simulink model "controlP"  (R2021a)
settings: Solver=VariableStepAuto  StartTime=0.0  StopTime=10.0  RelTol=1e-3
libraries: simulink x1
settings Model: Creator=phcs  LastModifiedBy=phcs

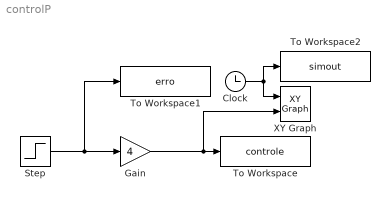
== system controlP ==
  Clock : Clock
  Gain : Gain  Gain=4
  Step : Step  Time=0  SampleTime=0
  To Workspace : ToWorkspace  VariableName=controle  SaveFormat=Timeseries  SampleTime=-1
  To Workspace1 : ToWorkspace  VariableName=erro  SaveFormat=Timeseries  SampleTime=-1
  To Workspace2 : ToWorkspace  VariableName=simout  SaveFormat=Timeseries  SampleTime=-1
  XY Graph : simulink/Sinks/XY Graph  xmin=0  xmax=10  ymin=0  ymax=5  st=-1
  wires:
  Step/1 -> To Workspace1/1, Gain/1
  Gain/1 -> XY Graph/2, To Workspace/1
  Clock/1 -> To Workspace2/1, XY Graph/1
